simulink model "OFDM_Reception_MessageHello"  (R2020b)
settings: Solver=VariableStepDiscrete  StartTime=0.0  StopTime=(660*10+66*2)*20e-6  RelTol=1e-3
PreLoadFcn:
  | N = 64;
  | TsOFDM = 3.2e-6;
  | nb_pilotes = 16;
  | sample_time = TsOFDM/(2*N);
  | nb_pc = 2;
InitFcn:
  | N = 64;
  | TsOFDM = 20e-6;
  | nb_pilotes = 16;
  | sample_time = TsOFDM/(2*N);
  | nb_pc = 2;
libraries: dspindex x6, commutil2 x1, commsink2 x1, dspxfrm3 x1, commdigbbndpm3 x1
settings Model: Creator=t_issarni  LastModifiedBy=t_issarni
settings DataIOCC: LimitDataPoints=on  SaveOutput=off  SaveTime=off
settings OptimizationCC: BooleanDataType=off  DefaultParameterBehavior=Inlined  LocalBlockOutputs=off  LifeSpan=inf
settings DebuggingCC: AlgebraicLoopMsg=error  SingleTaskRateTransMsg=error  AllowSymbolicDim=off  SFUnexpectedBacktrackingDiag=warning  SFNoUnconditionalDefaultTransitionDiag=warning  SFExecutionAtInitializationDiag=none  ArithmeticOperatorsInVariantConditions=warning
settings SFSimCC: SimUseLocalCustomCode=off  CustomCodeUndefinedFunction=UseInterfaceOnly
settings RTWCC: RTWUseLocalCustomCode=off
settings CodeAppCC: StateflowObjectComments=on
settings GRTTargetCC: TargetLangStandard=C89/C90 (ANSI)
settings ConfigComp: CovMetricSettings=dw  CovSaveCumulativeToWorkspaceVar=on  CovSaveSingleToWorkspaceVar=on  CovExternalEMLEnable=off  CovSFcnEnable=off

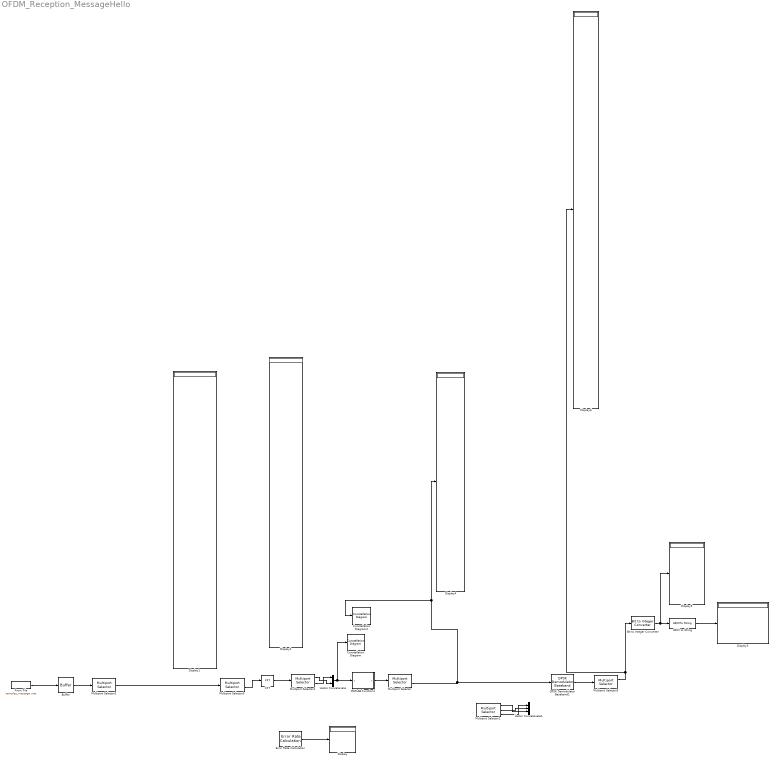
== system OFDM_Reception_MessageHello ==
  ASCII to String : ASCIIToString
  Bit to Integer Converter : commutil2/Bit to Integer Converter  nbits=8  bitOrder=MSB first  signedOutputValues=Unsigned  outDtype=uint8  outDtypeSigned=Inherit via internal rule
  Buffer : Buffer  N=660  OutputFrames=off
  Constellation Diagram : ConstellationDiagram
  Constellation Diagram2 : ConstellationDiagram
  Display{,1..6} (7 alike) : Display
  Error Rate Calculation : commsink2/Error Rate Calculation  N=0  st_delay=0  cp_mode=Entire frame  subframe=[]  PMode=Port  WsName=ErrorVec  RsMode2=off  stop=off  numErr=100  maxBits=1e6
      settings: SourceProductName=Communications Toolbox
  FFT : dspxfrm3/FFT  FFTImplementation=Auto  CompMethod=Table lookup  TableOpt=NEW  TableOptActive=Speed  BitRevOrder=off  Normalize=off  InheritFFTLength=on  FFTLength=64  WrapInput=on  roundingMode=Floor  overflowMode=off  firstCoeffDataTypeStr=Inherit: Same word length as input  firstCoeffLastDataTypeStr=Inherit: Same word length as input  outputMin=[]  outputMax=[]
  From File : FromFile  FileName=samples_message.mat  SampleTime=20e-6
  MATLAB Function1 : MATLAB Function  TreatAsAtomicUnit=on
  Multiport Selector : dspindex/Multiport Selector  rowsOrCols=Rows  idxCellArray={ 1, 2 : 48}  idxErrMode=Clip Index
  Multiport Selector1 : dspindex/Multiport Selector  rowsOrCols=Rows  idxCellArray="{1 : (N-nb_pilotes-nb_pc)/2,  (N-nb_pilotes-nb_pc)/2+1 ,  ((N-nb_pilotes-nb_pc)/2) + 2 : N-nb_pilotes-nb_pc+1}"  idxErrMode=Clip Index
  Multiport Selector2 : dspindex/Multiport Selector  rowsOrCols=Rows  idxCellArray={ 1:66, 67 : 132 , 133: 660 }  idxErrMode=Clip Index
  Multiport Selector3 : dspindex/Multiport Selector  rowsOrCols=Rows  idxCellArray="{1 : 2,  3 : 66}"  idxErrMode=Clip Index
  Multiport Selector4 : dspindex/Multiport Selector  rowsOrCols=Rows  idxCellArray={1:32, 33: 64}  idxErrMode=Clip Index
  Multiport Selector5 : dspindex/Multiport Selector  rowsOrCols=Rows  idxCellArray={1 : 88 , 89 : 94}  idxErrMode=Clip Index
  QPSK Demodulator Baseband1 : commdigbbndpm3/QPSK Demodulator Baseband  OutType=Bit  DecType=Hard decision  VarSource=Dialog  Variance=1  Dec=Gray  Ph=pi/4  outDtype1=Inherit via internal rule  outDtype2=Inherit via internal rule  derotateFactorWordLen=16  derotateFactorDataTypeStr=Inherit: Same word length as input  derotateFactorLastDataTypeStr=Inherit: Same word length as input
      settings: SourceProductName=Communications Toolbox
  Vector Concatenate : Concatenate
  Vector Concatenate1 : Concatenate  NumInputs=3
  wires:
  Error Rate Calculation/1 -> Display/1
  Multiport Selector3/2 -> FFT/1
  QPSK Demodulator Baseband1/1 -> Multiport Selector5/1
  Bit to Integer Converter/1 -> Display5/1, ASCII to String/1
  Multiport Selector5/1 -> Bit to Integer Converter/1, Display6/1
  ASCII to String/1 -> Display3/1
  From File/1 -> Buffer/1
  Multiport Selector1/1 -> Vector Concatenate1/3
  Multiport Selector1/3 -> Vector Concatenate1/1
  Multiport Selector1/2 -> Vector Concatenate1/2
  MATLAB Function1/1(y) -> Multiport Selector/1
  Multiport Selector/2 -> QPSK Demodulator Baseband1/1, Constellation Diagram2/1, Display4/1
  Buffer/1 -> Multiport Selector2/1
  Multiport Selector2/2 -> Multiport Selector3/1
  Multiport Selector4/2 -> Vector Concatenate/1
  Multiport Selector4/1 -> Vector Concatenate/2
  FFT/1 -> Multiport Selector4/1
  Vector Concatenate/1 -> MATLAB Function1/1(x), Constellation Diagram/1

== matlab function OFDM_Reception_MessageHello/MATLAB Function1 ==
  data: x input; y output; nb_pilotes parameter; N parameter; nb_pc parameter
function y = fcn(x, nb_pilotes, N, nb_pc)
d= 48;
y = complex(zeros(d,1));
samples_out = complex(zeros(d,1));
samples = complex(zeros(d,1));
pilotes = complex(zeros(nb_pilotes,1));
pas = ceil((N-nb_pc)/nb_pilotes);
x_retourne = complex(zeros(64,1));
samples_out_retourne = complex(zeros(d,1));




last_idx_pilote = 1;
last_idx_sample = 1; 


% inversion de l'échantillion 
for i = 1 : 64
    x_retourne(i,1) = complex(x(65 - i,1));
end 

% on sépare les pilotes et les échantillons
for i=1:d + nb_pilotes
    if mod(i-1,pas) == 0 || last_idx_sample > d
        pilotes(last_idx_pilote, 1) = x_retourne(i,1);
        last_idx_pilote = last_idx_pilote +1;

    else      
        samples(last_idx_sample, 1) = complex(x_retourne(i,1));
        last_idx_sample = last_idx_sample +1;
    end
end



nb_samples_parcouru = 0;
pilotes_parcouru = 0;
for i=1:nb_pilotes 
    
    ecart = pas;
    
    
    if nb_samples_parcouru >= d - (pas-1)    
        ecart = 47 - nb_samples_parcouru + 1;
    end

    
    if pilotes_parcouru < nb_pilotes - 1 
        pente_RE = (real(pilotes(pilotes_parcouru + 2, 1)) - real(pilotes(pilotes_parcouru + 1, 1))) / ecart;
        pente_IM = (imag(pilotes(pilotes_parcouru + 2, 1)) - imag(pilotes(pilotes_parcouru + 1, 1))) / ecart;
        temps = 0:ecart;
        equation_pente_real = pente_RE*temps + real(pilotes(pilotes_parcouru + 1, 1));
        equation_pente_imag = pente_IM*temps + imag(pilotes(pilotes_parcouru + 1, 1));
        coef_interpo = complex(zeros(ecart+1,1));

        % calcul coefficients d'interpolation
        for p=1:ecart+1
            coef_interpo(p,1) = complex(equation_pente_real(1,p), equation_pente_imag(1,p));
        end
        
       
        for j=1:pas-1
            % calcul interpolation
            if nb_samples_parcouru < d
                samples_out((i-1)*(pas-1) + j,1) = samples((i-1)*(pas-1) + j,1) / coef_interpo(j+1,1);
                nb_samples_parcouru = nb_samples_parcouru + 1;
            end

        end
       
    else
        for j=1:pas-1
                if nb_samples_parcouru < d
                    samples_out((i-1)*(pas-1) + j,1) = samples((i-1)*(pas-1) + j,1) / pilotes(16,1);
                    nb_samples_parcouru = nb_samples_parcouru + 1;
                end
        end
    end 
    
    pilotes_parcouru = pilotes_parcouru + 1;
end

for i = 1 : 48
    samples_out_retourne(i, 1) = samples_out(49 - i,1);
end 


y = samples_out_retourne;





% 
% % on calcule la phase et le module de chaque échantillon
% for i=1:N-nb_pilotes-nb_pc
%     modules(i,1) = abs(samples_out(i,1));
%     phases(i,1) = angle(samples_out(i,1));
% end


% compteur = 1;
% pilotes_parcouru = 0;
% nb_samples_parcouru = 0;
% for i=1:nb_pilotes - 1
%     
% %     if pilotes_parcouru < nb_pilotes - 1 
%         ecart = pas;
%         if nb_samples_parcouru >= N-nb_pilotes-nb_pc - (pas-1)
%             ecart = N-nb_pilotes-nb_pc - nb_samples_parcouru + 1;
%         end
%         
%         pente_module = (abs(pilotes(pilotes_parcouru + 2, 1)) - abs(pilotes(pilotes_parcouru + 1, 1))) / ecart;
%         pente_phase = (angle(pilotes(pilotes_parcouru + 2, 1)) - angle(pilotes(pilotes_parcouru + 1, 1))) / ecart;
%         
%         x = 0:ecart;
%         equation_pente_module = pente_module*x + abs(pilotes(pilotes_parcouru + 1, 1));
%         equation_pente_phase = pente_phase*x + angle(pilotes(pilotes_parcouru + 1, 1));
%         
%         
%         for j=1:pas-1
%             % calcul sur chaque coeff
%             if nb_samples_parcouru < N-nb_pilotes-nb_pc
%                 coef_IL_mod(compteur,1) = modules((pilotes_parcouru * (pas-1)) + j,1) / equation_pente_module(1,j+1);
%                 coef_IL_phase(compteur,1) = phases((pilotes_parcouru * (pas-1)) + j,1) - equation_pente_phase(1,j+1);
%                 nb_samples_parcouru = nb_samples_parcouru + 1;
%             end
%             
%             compteur = compteur + 1;
%         end
%         
%         pilotes_parcouru = pilotes_parcouru + 1;
%         
%         
% %     else
% %         % pente constante
% %         pente_module = abs(pilotes(pilotes_parcouru, 1));
% %         pente_phase = angle(pilotes(pilotes_parcouru, 1));
% %         for j=1:pas-1
% %             % calcul sur chaque coeff
% %             disp('____________-')
% %             coef_IL_mod(compteur,1) = modules((pilotes_parcouru * (pas-1)) + j,1) / pente_module;
% %             disp(coef_IL_mod(compteur,1))
% %             coef_IL_phase(compteur,1) = phases((pilotes_parcouru * (pas-1)) + j,1) - pente_phase;
% %             disp(coef_IL_phase(compteur,1))
% %             compteur = compteur + 1;
% %         end
% %         
% %     end
%  
% end
% 
% 
% % on assemble partie réelle et imaginaire
% for j=1:N-nb_pilotes-nb_pc
%     
%     if (modules(j,1) && phases(j,1)) ~= 0
%         samples_out(j,1) = coef_IL_mod(j,1)*(cos(coef_IL_phase(j,1)) + complex(0,1)* sin(coef_IL_phase(j,1)));
%     else
%         samples_out(j,1) = 0;
%     end
%     
% end
% 
% 
% %
% % compteur_tour = 1;
% % for i=1:nb_pilotes
% %     for j=1:pas
% %         if i == nb_pilotes 
% %             if compteur_tour > size(coef_IL_mod)
% %                break
% %             else 
% %                 disp("hello");
% %                 coef_IL_mod(compteur_tour, 1) = modules(i,1);
% %                 coef_IL_phase(compteur_tour, 1) = phases(i,1);
% %                 disp(coef_IL_mod(compteur_tour, 1));
% %                 compteur_tour = compteur_tour + 1;
% %             end
% %         else 
% %             disp(compteur_tour);
% %             coef_IL_mod(compteur_tour, 1) = modules(i,1) + ((modules(i+1,1)-modules(i,1))/(pas-2))*(j-1);
% %             coef_IL_phase(compteur_tour, 1) = phases(i,1) + ((phases(i+1,1)-phases(i,1))/(pas-2))*(j-1);
% % 
% %             disp((modules(i+1,1)-modules(i,1))/(pas-1));
% %             compteur_tour = compteur_tour + 1;
% %         end 
% %     end
% % end
% % 
% % 
% % for i=1:compteur_tour-1
% %     disp(coef_IL_mod(i,1));
% %     samples_out(i, 1) = (samples_out(i, 1) / coef_IL_mod(i, 1));
% % end
% % 
% 
% %4*(TsOFDM/N)
